simulink model "RK_T11_d"  (R2016a)
settings: Solver=ode45  StartTime=0.0  StopTime=25  RelTol=1e-3
model workspace (MATLAB code in the model file):
  | Ks = 1.5;
  | T = 1.73; % s
  | D = 1.15;
  | % - - - - - - - - - - -
  | d = 1;  % diskrete Laufzeit
  | % - - - - - - - - - - -
  | Tg = 5.2; % s
  | T0 = 0.25; % s
  | Tu = 0.45+T0*d; % s
  | % - - - - - - - - - - -
  | Kp = 1.2*Tg/Ks/(Tu+T0);
  | Tv = (Tu+T0)/2; % s
  | Tn = 2*(Tu+T0/2)^2/(Tu+T0); % s
  | % - - - - - - - - - - -
  | p1 = -1;
  | q0 = Kp*(1+T0/2/Tn+Tv/T0);
  | q1 = -Kp*(1-T0/2/Tn+2*Tv/T0);
  | q2 = Kp*Tv/T0;
Description:
  | Regelkreis mit kontinuierlichem PID-Regler
settings Model: ExtModeAutoUpdateStatusClock=off  Creator=manfred  LastModifiedBy=manfred
settings DataIOCC: LimitDataPoints=on  SaveFormat=Array  SignalLoggingSaveFormat=ModelDataLogs  SignalLoggingName=sigsOut
settings OptimizationCC: ExpressionDepthLimit=2147483647
settings DebuggingCC: SaveWithParameterizedLinksMsg=none  UnderspecifiedInitializationDetection=Classic  MergeDetectMultiDrivingBlocksExec=none  SignalResolutionControl=TryResolveAllWithWarning  MultiTaskDSMMsg=warning  MultiTaskCondExecSysMsg=none  FcnCallInpInsideContextMsg=UseLocalSettings  StateNameClashWarn=warning  StrictBusMsg=None
settings HardwareCC: ProdBitPerPointer=32  ProdLargestAtomicFloat=None  ProdIntDivRoundTo=Undefined  ProdEndianess=Unspecified  ProdWordSize=32  ProdHWDeviceType=32-bit Generic  TargetUnknown=on
settings ModelReferenceCC: PropagateSignalLabelsOutOfModel=off
settings GRTTargetCC: GeneratePreprocessorConditionals=Use local settings  CombineOutputUpdateFcns=off  GRTInterface=on
settings ConfigComp: CovModelRefEnable=Off

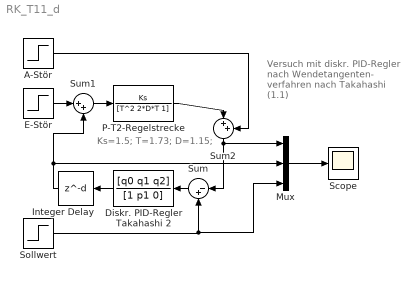
== system RK_T11_d ==
  note: Ks=1.5; T=1.73; D=1.15;
  note: Versuch mit diskr.
      | PID-Regler nach
      | Wendetangenten-
      | verfahren nach
      | Takahashi (1.1)
  A-Stör : Step  Time=15  SampleTime=0
  Diskr. PID-Regler Takahashi 2 : DiscreteTransferFcn  Numerator=[q0 q1 q2]  Denominator=[1 p1 0]  SampleTime=T0
  E-Stör : Step  Time=8  SampleTime=0
  Integer Delay : Delay  DelayLength=d  InputProcessing=Inherited
  Mux : Mux  Inputs=3
  P-T2-Regelstrecke : TransferFcn  Numerator=Ks  Denominator=[T^2 2*D*T 1]  ContinuousStateAttributes='Regelstrecke'
  Scope : Scope
  Sollwert : Step  SampleTime=0
  Sum : Sum  Inputs=|-+  SaturateOnIntegerOverflow=on
  Sum1 : Sum  Inputs=|++
  Sum2 : Sum  Inputs=|++
  wires:
  Mux/1 -> Scope/1
  Sum1/1 -> P-T2-Regelstrecke/1
  Sum2/1 -> Sum/1, Mux/1
  P-T2-Regelstrecke/1 -> Sum2/1
  Sollwert/1 -> Mux/3, Sum/2
  E-Stör/1 -> Sum1/1
  A-Stör/1 -> Sum2/2
  Sum/1 -> Diskr. PID-Regler Takahashi 2/1
  Diskr. PID-Regler Takahashi 2/1 -> Integer Delay/1
  Integer Delay/1 -> Sum1/2, Mux/2
